simulink model "a621"  (R2019b)
settings: Solver=VariableStepAuto  StartTime=0.0  StopTime=300.0  RelTol=1e-3
settings Model: Creator=ovi  LastModifiedBy=ovi

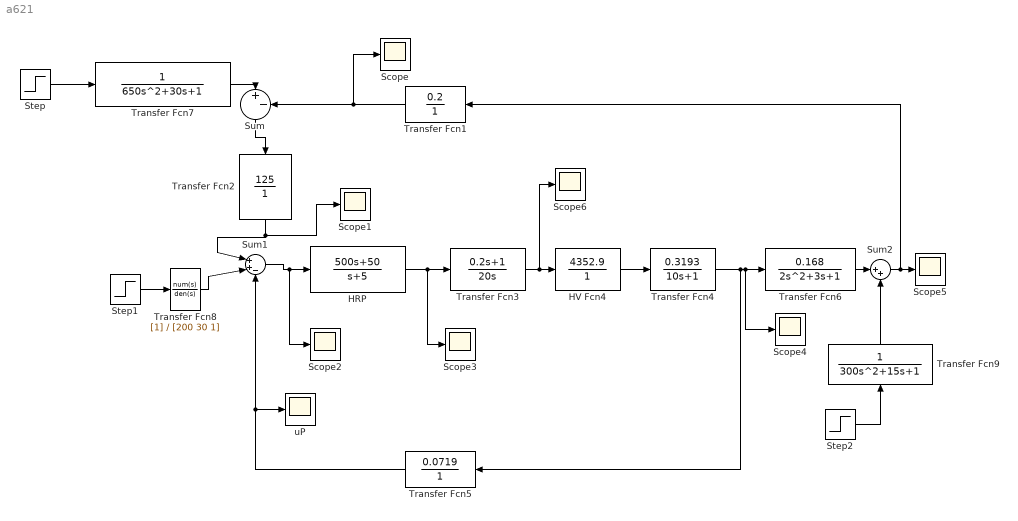
== system a621 ==
  " HV Fcn4" : TransferFcn  Numerator=[4352.9]  Denominator=[1]
  HRP : TransferFcn  Numerator=[500 50]  Denominator=[1 5]
  Scope{,1..6} (7 alike) : Scope
  Step : Step  After=10  SampleTime=0
  Step1 : Step  After=10  SampleTime=0
  Step2 : Step  Time=150  After=-1  SampleTime=0
  Sum : Sum  Inputs=|+-
  Sum1 : Sum  Inputs=|++-
  Sum2 : Sum  Inputs=|++
  Transfer Fcn1 : TransferFcn  Numerator=[0.2]  Denominator=[1]
  Transfer Fcn2 : TransferFcn  Numerator=[125]  Denominator=[1]
  Transfer Fcn3 : TransferFcn  Numerator=[0.2 1]  Denominator=[20 0]
  Transfer Fcn4 : TransferFcn  Numerator=[0.3193]  Denominator=[10 1]
  Transfer Fcn5 : TransferFcn  Numerator=[0.0719]  Denominator=[1]
  Transfer Fcn6 : TransferFcn  Numerator=0.168  Denominator=[2 3 1]
  Transfer Fcn7 : TransferFcn  Denominator=[650 30 1]
  Transfer Fcn8 : TransferFcn  Denominator=[200 30 1]
  Transfer Fcn9 : TransferFcn  Denominator=[300 15 1]
  uP : Scope
  wires:
  Step/1 -> Transfer Fcn7/1
  Transfer Fcn1/1 -> Scope/1, Sum/2
  Sum/1 -> Transfer Fcn2/1
  Transfer Fcn2/1 -> Scope1/1, Sum1/1
  Step1/1 -> Transfer Fcn8/1
  Sum1/1 -> Scope2/1, HRP/1
  HRP/1 -> Scope3/1, Transfer Fcn3/1
  Transfer Fcn3/1 -> Scope6/1, " HV Fcn4"/1
  " HV Fcn4"/1 -> Transfer Fcn4/1
  Transfer Fcn4/1 -> Transfer Fcn5/1, Scope4/1, Transfer Fcn6/1
  Transfer Fcn5/1 -> uP/1, Sum1/3
  Transfer Fcn6/1 -> Sum2/1
  Step2/1 -> Transfer Fcn9/1
  Sum2/1 -> Transfer Fcn1/1, Scope5/1
  Transfer Fcn7/1 -> Sum/1
  Transfer Fcn8/1 -> Sum1/2
  Transfer Fcn9/1 -> Sum2/2
